simulink model "Motor_Position_contol_system"  (R2020b)
settings: Solver=ode14x  StartTime=0.0  StopTime=10.0  FixedStep=0.1  RelTol=1e-3
values from neighbouring files (symbols this model uses):
  b = 3.5077E-6    [datadic.sldd]
  J = 3.2284E-6    [datadic.sldd]
  K = 0.0274    [datadic.sldd]
  kd = 0.13907    [datadic.sldd]
  ki = 523.2955    [datadic.sldd]
  kp = 17.3682    [datadic.sldd]
  L = 2.75E-6    [datadic.sldd]
  R = 4.0    [datadic.sldd]
settings Model: Creator=ARPITA  LastModifiedBy=ARPITA
settings DataIOCC: SaveOutput=off  SaveTime=off

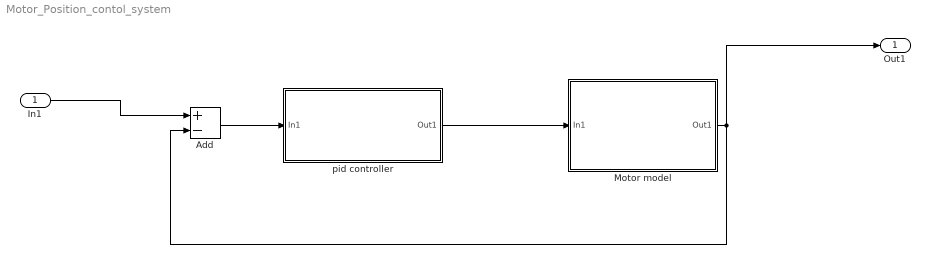
== system Motor_Position_contol_system ==
  In1 : Inport  OutDataTypeStr=double  PortDimensions=1  SampleTime=0
  Add : Sum  Inputs=+-
  Motor model : Subsystem
  pid controller : Subsystem
  Out1 : Outport  OutDataTypeStr=double  PortDimensions=1  SampleTime=0
  wires:
  Motor model/1(Out1) -> Add/2, Out1/1
  In1/1 -> Add/1
  Add/1 -> pid controller/1(In1)
  pid controller/1(Out1) -> Motor model/1(In1)

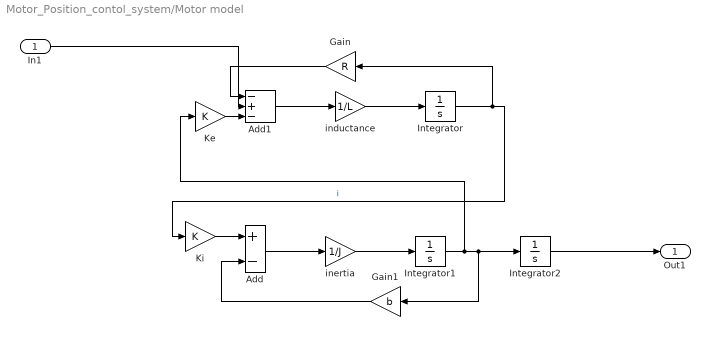
== system Motor_Position_contol_system/Motor model ==
  In1 : Inport
  Add : Sum  Inputs=+-
  Add1 : Sum  Inputs=-+-
  Gain : Gain  Gain=R
  Gain1 : Gain  Gain=b
  Integrator : Integrator
  Integrator1 : Integrator
  Integrator2 : Integrator
  Ke : Gain  Gain=K
  Ki : Gain  Gain=K
  inductance : Gain  Gain=1/L
  inertia : Gain  Gain=1/J
  Out1 : Outport
  wires:
  inductance/1 -> Integrator/1
  In1/1 -> Add1/2
  Ki/1 -> Add/1
  Gain/1 -> Add1/1
  Integrator2/1 -> Out1/1
  Integrator/1 -> Gain/1, Ki/1  "i"
  Add1/1 -> inductance/1
  inertia/1 -> Integrator1/1
  Ke/1 -> Add1/3
  Integrator1/1 -> Ke/1, Gain1/1, Integrator2/1
  Add/1 -> inertia/1
  Gain1/1 -> Add/2

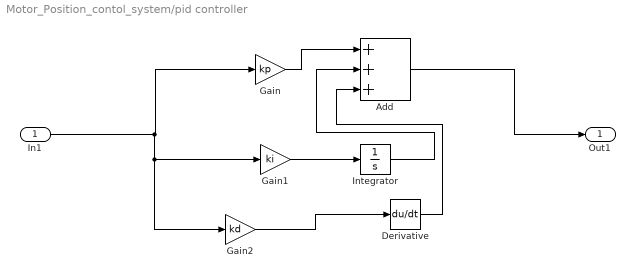
== system Motor_Position_contol_system/pid controller ==
  In1 : Inport
  Add : Sum  Inputs=+++
  Derivative : Derivative
  Gain : Gain  Gain=kp
  Gain1 : Gain  Gain=ki
  Gain2 : Gain  Gain=kd
  Integrator : Integrator
  Out1 : Outport
  wires:
  Derivative/1 -> Add/3
  Integrator/1 -> Add/2
  Gain2/1 -> Derivative/1
  Add/1 -> Out1/1
  In1/1 -> Gain/1, Gain2/1, Gain1/1
  Gain/1 -> Add/1
  Gain1/1 -> Integrator/1
